simulink model "testModel"  (R2021b)
settings: Solver=VariableStepAuto  StartTime=0.0  StopTime=5  RelTol=1e-3
undefined symbols (not defined in the file): den, num
libraries: slpidlib x2
settings Model: Creator=mobil  LastModifiedBy=mobil

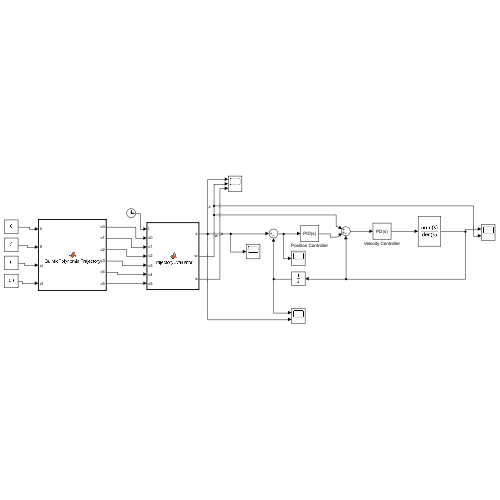
[thumbnail: Simulink's stored preview of the top-level diagram]
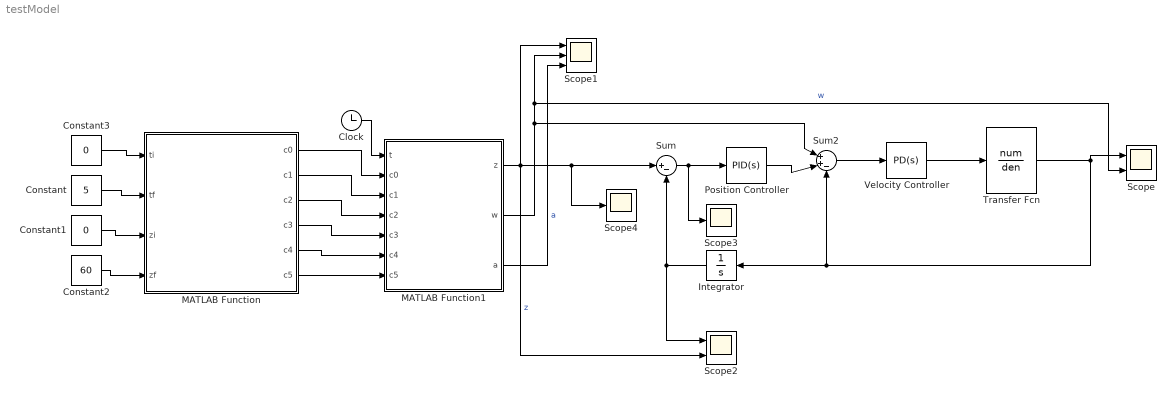
== system testModel ==
  Clock : Clock
  Constant : Constant  Value=5
  Constant1 : Constant  Value=0
  Constant2 : Constant  Value=60
  Constant3 : Constant  Value=0
  Integrator : Integrator
  MATLAB Function : MATLAB Function  TreatAsAtomicUnit=on
  MATLAB Function1 : MATLAB Function  TreatAsAtomicUnit=on
  Position Controller : slpidlib/PID Controller  Controller=PID  Form=Parallel  TimeDomain=Continuous-time  UseExternalTs=off  SampleTime=-1  IntegratorMethod=Forward Euler  FilterMethod=Forward Euler  ControllerParametersSource=internal  P=395.429721379344  I=11710.7973359679  D=3.30901436747134  UseFilter=on  N=34048.4681165414  TunerSelectOption=Transfer Function Based (PID Tuner App)  InitialConditionSource=internal  InitialConditionForIntegrator=0  InitialConditionForFilter=0  DifferentiatorICPrevScaledInput=0  ExternalReset=none  TrackingMode=off  Kt=1  LimitOutput=off  SatLimitsSource=internal  UpperSaturationLimit=inf  LowerSaturationLimit=-inf  LinearizeAsGain=on  AntiWindupMode=none  Kb=1  POutMin=[]  POutMax=[]  IOutMin=[]  IOutMax=[]  DOutMin=[]  DOutMax=[]  NOutMin=[]  NOutMax=[]  SumOutMin=[]  SumOutMax=[]  SaturationOutMin=[]  SaturationOutMax=[]  PParamMin=[]  PParamMax=[]  IParamMin=[]  IParamMax=[]  DParamMin=[]  DParamMax=[]  NParamMin=[]  NParamMax=[]  KbParamMin=[]  KbParamMax=[]  KtParamMin=[]  KtParamMax=[]  KbOutMin=[]  KbOutMax=[]  KtOutMin=[]  KtOutMax=[]  IntegratorOutMin=[]  IntegratorOutMax=[]  FilterOutMin=[]  FilterOutMax=[]  SumI1OutMin=[]  SumI1OutMax=[]  SumI2OutMin=[]  SumI2OutMax=[]  SumI3OutMin=[]  SumI3OutMax=[]  SumI4OutMin=[]  SumI4OutMax=[]  SumDOutMin=[]  SumDOutMax=[]  DifferentiatorOutMin=[]  DifferentiatorOutMax=[]  FilterDiffOutCoefMin=[]  FilterDiffOutCoefMax=[]  ReciprocalOutMin=[]  ReciprocalOutMax=[]  SumDenOutMin=[]  SumDenOutMax=[]  SumNumOutMin=[]  SumNumOutMax=[]  DivideOutMin=[]  DivideOutMax=[]  UdiffTsProdOutMin=[]  UdiffTsProdOutMax=[]  NTsProdOutMin=[]  NTsProdOutMax=[]  UintegralTsProdOutMin=[]  UintegralTsProdOutMax=[]  UngainTsProdOutMin=[]  UngainTsProdOutMax=[]  IntegratorContinuousStateAttributes=''  IntegratorStateMustResolveToSignalObject=off  IntegratorRTWStateStorageClass=Auto  FilterContinuousStateAttributes=''  FilterStateMustResolveToSignalObject=off  FilterRTWStateStorageClass=Auto  ParallelPVariant=InternalParameters  IdealPVariant=Disabled  IVariant=InternalParameters  DVariant=InternalParameters  IntegratorVariant=Continuous  SatVariant=Disabled  AWVariant=Passthrough  PCopyVariant=Disabled  TRVariant=Disabled  FdbkBlocksVariant=Forward  IdealPFdbkVariant=Disabled  SatFdbkVariant=Disabled  DerivativeFilterVariant=ContFilter  NVariant=InternalParameters  NCopyVariant=Disabled  FilterICVariant=InternalICsFilter  IntegratorICVariant=InternalICs  ExternalResetVariant=Disabled  TRSumVariant=Passthrough  SumFdbkVariant=Disabled  SumVariant=Sum_PID  TsampFilterVariant=InternalTs  TsampNgainVariant=Passthrough  TsampIntegralVariant=Passthrough  ExternalSaturationOutDataTypeStr=Inherit: Same as second input
  Scope : Scope  NumInputPorts=2
  Scope1 : Scope  NumInputPorts=3
  Scope2 : Scope  NumInputPorts=2
  Scope3 : Scope
  Scope4 : Scope
  Sum : Sum  Inputs=|+-
  Sum2 : Sum  Inputs=|++-
  Transfer Fcn : TransferFcn  Numerator=num  Denominator=den
  Velocity Controller : slpidlib/PID Controller  Controller=PD  Form=Parallel  TimeDomain=Continuous-time  UseExternalTs=off  SampleTime=-1  IntegratorMethod=Forward Euler  FilterMethod=Forward Euler  ControllerParametersSource=internal  P=4.75285728911875  I=0  D=0.0552140472497039  UseFilter=on  N=12501.0342930318  TunerSelectOption=Transfer Function Based (PID Tuner App)  InitialConditionSource=internal  InitialConditionForIntegrator=0  InitialConditionForFilter=0  DifferentiatorICPrevScaledInput=0  ExternalReset=none  TrackingMode=off  Kt=1  LimitOutput=off  SatLimitsSource=internal  UpperSaturationLimit=inf  LowerSaturationLimit=-inf  LinearizeAsGain=on  AntiWindupMode=none  Kb=1  POutMin=[]  POutMax=[]  IOutMin=[]  IOutMax=[]  DOutMin=[]  DOutMax=[]  NOutMin=[]  NOutMax=[]  SumOutMin=[]  SumOutMax=[]  SaturationOutMin=[]  SaturationOutMax=[]  PParamMin=[]  PParamMax=[]  IParamMin=[]  IParamMax=[]  DParamMin=[]  DParamMax=[]  NParamMin=[]  NParamMax=[]  KbParamMin=[]  KbParamMax=[]  KtParamMin=[]  KtParamMax=[]  KbOutMin=[]  KbOutMax=[]  KtOutMin=[]  KtOutMax=[]  IntegratorOutMin=[]  IntegratorOutMax=[]  FilterOutMin=[]  FilterOutMax=[]  SumI1OutMin=[]  SumI1OutMax=[]  SumI2OutMin=[]  SumI2OutMax=[]  SumI3OutMin=[]  SumI3OutMax=[]  SumI4OutMin=[]  SumI4OutMax=[]  SumDOutMin=[]  SumDOutMax=[]  DifferentiatorOutMin=[]  DifferentiatorOutMax=[]  FilterDiffOutCoefMin=[]  FilterDiffOutCoefMax=[]  ReciprocalOutMin=[]  ReciprocalOutMax=[]  SumDenOutMin=[]  SumDenOutMax=[]  SumNumOutMin=[]  SumNumOutMax=[]  DivideOutMin=[]  DivideOutMax=[]  UdiffTsProdOutMin=[]  UdiffTsProdOutMax=[]  NTsProdOutMin=[]  NTsProdOutMax=[]  UintegralTsProdOutMin=[]  UintegralTsProdOutMax=[]  UngainTsProdOutMin=[]  UngainTsProdOutMax=[]  IntegratorContinuousStateAttributes=''  IntegratorStateMustResolveToSignalObject=off  IntegratorRTWStateStorageClass=Auto  FilterContinuousStateAttributes=''  FilterStateMustResolveToSignalObject=off  FilterRTWStateStorageClass=Auto  ParallelPVariant=InternalParameters  IdealPVariant=Disabled  IVariant=Disabled  DVariant=InternalParameters  IntegratorVariant=Disabled  SatVariant=Disabled  AWVariant=Disabled  PCopyVariant=Disabled  TRVariant=Disabled  FdbkBlocksVariant=Forward  IdealPFdbkVariant=Disabled  SatFdbkVariant=Disabled  DerivativeFilterVariant=ContFilter  NVariant=InternalParameters  NCopyVariant=Disabled  FilterICVariant=InternalICsFilter  IntegratorICVariant=Disabled  ExternalResetVariant=Disabled  TRSumVariant=Passthrough  SumFdbkVariant=Disabled  SumVariant=Sum_PD  TsampFilterVariant=InternalTs  TsampNgainVariant=Passthrough  TsampIntegralVariant=Disabled_SignalSpec  ExternalSaturationOutDataTypeStr=Inherit: Same as second input
  wires:
  Constant3/1 -> MATLAB Function/1(ti)
  Constant/1 -> MATLAB Function/2(tf)
  Constant1/1 -> MATLAB Function/3(zi)
  Constant2/1 -> MATLAB Function/4(zf)
  MATLAB Function1/1(z) -> Scope1/1, Scope2/2, Scope4/1, Sum/1  "z"
  Clock/1 -> MATLAB Function1/1(t)
  MATLAB Function/1(c0) -> MATLAB Function1/2(c0)
  MATLAB Function/2(c1) -> MATLAB Function1/3(c1)
  MATLAB Function/3(c2) -> MATLAB Function1/4(c2)
  MATLAB Function/4(c3) -> MATLAB Function1/5(c3)
  MATLAB Function/5(c4) -> MATLAB Function1/6(c4)
  MATLAB Function/6(c5) -> MATLAB Function1/7(c5)
  MATLAB Function1/2(w) -> Scope1/2, Scope/2, Sum2/1  "w"
  MATLAB Function1/3(a) -> Scope1/3  "a"
  Sum/1 -> Scope3/1, Position Controller/1
  Velocity Controller/1 -> Transfer Fcn/1
  Transfer Fcn/1 -> Integrator/1, Sum2/3, Scope/1
  Integrator/1 -> Scope2/1, Sum/2
  Sum2/1 -> Velocity Controller/1
  Position Controller/1 -> Sum2/2

== matlab function testModel/MATLAB Function1 ==
  data: t input; z output; c0 input; w output; a output; c1 input; c2 input; c3 input; c4 input; c5 input
function [z,w,a] = TrajectoryEvaluator(t,c0,c1,c2,c3,c4,c5)
    z = c0+c1*t+c2*t^2+c3*t^3+c4*t^4+c5*t^5;
    w = c1+2*c2*t+3*c3*t^2+4*c4*t^3+5*c5*t^4;
    a = 2*c2+6*c3*t+12*c4*t^2+20*c5*t^3;
;

== matlab function testModel/MATLAB Function ==
  data: ti input; c0 output; tf input; zi input; zf input; c1 output; c2 output; c3 output; c4 output; c5 output
function [c0,c1,c2,c3,c4,c5] = QuinticPolynomialTrajectory(ti,tf,zi,zf)
%#codegen
    wi = 0;
    ai = 0;
    wf = 0;
    af = 0;
    c0 = (2*tf^5*zi - 2*ti^5*zf + 2*tf*ti^5*wf - 2*tf^5*ti*wi + 10*tf*ti^4*zf - 10*tf^4*ti*zi - af*tf^2*ti^5 + 2*af*tf^3*ti^4 - af*tf^4*ti^3 + ai*tf^3*ti^4 - 2*ai*tf^4*ti^3 + ai*tf^5*ti^2 - 10*tf^2*ti^4*wf + 8*tf^3*ti^3*wf - 8*tf^3*ti^3*wi + 10*tf^4*ti^2*wi - 20*tf^2*ti^3*zf + 20*tf^3*ti^2*zi)/(2*(tf - ti)^2*(tf^3 - 3*tf^2*ti + 3*tf*ti^2 - ti^3));
    c1 = (2*tf^5*wi - 2*ti^5*wf + 2*af*tf*ti^5 - 2*ai*tf^5*ti + 10*tf*ti^4*wf - 10*tf^4*ti*wi - af*tf^2*ti^4 - 4*af*tf^3*ti^3 + 3*af*tf^4*ti^2 - 3*ai*tf^2*ti^4 + 4*ai*tf^3*ti^3 + ai*tf^4*ti^2 + 16*tf^2*ti^3*wf - 24*tf^3*ti^2*wf + 24*tf^2*ti^3*wi - 16*tf^3*ti^2*wi + 60*tf^2*ti^2*zf - 60*tf^2*ti^2*zi)/(2*(tf - ti)^2*(tf^3 - 3*tf^2*ti + 3*tf*ti^2 - ti^3));
    c2 = -(af*ti^5 - ai*tf^5 + 4*af*tf*ti^4 + 3*af*tf^4*ti - 3*ai*tf*ti^4 - 4*ai*tf^4*ti + 36*tf*ti^3*wf - 24*tf^3*ti*wf + 24*tf*ti^3*wi - 36*tf^3*ti*wi + 60*tf*ti^2*zf + 60*tf^2*ti*zf - 60*tf*ti^2*zi - 60*tf^2*ti*zi - 8*af*tf^2*ti^3 + 8*ai*tf^3*ti^2 - 12*tf^2*ti^2*wf + 12*tf^2*ti^2*wi)/(2*(tf - ti)^2*(tf^3 - 3*tf^2*ti + 3*tf*ti^2 - ti^3));
    c3 = (af*tf^4 + 3*af*ti^4 - 3*ai*tf^4 - ai*ti^4 - 8*tf^3*wf - 12*tf^3*wi + 12*ti^3*wf + 8*ti^3*wi + 20*tf^2*zf - 20*tf^2*zi + 20*ti^2*zf - 20*ti^2*zi + 4*af*tf^3*ti - 4*ai*tf*ti^3 + 28*tf*ti^2*wf - 32*tf^2*ti*wf + 32*tf*ti^2*wi - 28*tf^2*ti*wi - 8*af*tf^2*ti^2 + 8*ai*tf^2*ti^2 + 80*tf*ti*zf - 80*tf*ti*zi)/(2*(tf^2 - 2*tf*ti + ti^2)*(tf^3 - 3*tf^2*ti + 3*tf*ti^2 - ti^3));
    c4 = -(30*tf*zf - 30*tf*zi + 30*ti*zf - 30*ti*zi + 2*af*tf^3 + 3*af*ti^3 - 3*ai*tf^3 - 2*ai*ti^3 - 14*tf^2*wf - 16*tf^2*wi + 16*ti^2*wf + 14*ti^2*wi - 4*af*tf*ti^2 - af*tf^2*ti + ai*tf*ti^2 + 4*ai*tf^2*ti - 2*tf*ti*wf + 2*tf*ti*wi)/(2*(tf - ti)^2*(tf^3 - 3*tf^2*ti + 3*tf*ti^2 - ti^3));
    c5 = (12*zf - 12*zi - 6*tf*wf - 6*tf*wi + 6*ti*wf + 6*ti*wi + af*tf^2 + af*ti^2 - ai*tf^2 - ai*ti^2 - 2*af*tf*ti + 2*ai*tf*ti)/(2*(tf^2 - 2*tf*ti + ti^2)*(tf^3 - 3*tf^2*ti + 3*tf*ti^2 - ti^3));
